simulink model "encoder"  (R2024b)
settings: Solver=FixedStepAuto  StartTime=0.0  StopTime=50  FixedStep=0.1  RelTol=1e-3  EnableMultiTasking=on
libraries: stm32f4xxblockslib x4, stm32g4xxblockslib x3, simulink x2
settings Model: STM32="{\"EncoderBlockForG4\":[{\"ID\":\"encoder:1\"},{\"ID\":\"encoder:3\"},{\"ID\":\"encoder:4\"}],\"DigitalPortRead\":[{\"ID\":\"encoder:8\"},{\"ID\":\"encoder:9\"},{\"ID\":\"encoder:25\"},{\"ID\":\"encoder:32\"}]}"  Creator=FREED  LastModifiedBy=FREED
settings OptimizationCC: DefaultParameterBehavior=Inlined  EnhancedBackFolding=on  PassReuseOutputArgsAs=Individual arguments  ZeroExternalMemoryAtStartup=off  ZeroInternalMemoryAtStartup=off  MaxStackSize=512  OptimizeBlockOrder=speed  DifferentSizesBufferReuse=on  OptimizationCustomize=off  EfficientTunableParamExpr=on
settings DebuggingCC: ParameterTunabilityLossMsg=error
settings HardwareCC: ProdBitPerPointer=32  ProdBitPerSizeT=32  ProdBitPerPtrDiffT=32  ProdLargestAtomicInteger=Long  ProdLargestAtomicFloat=Double  ProdWordSize=32  ProdLongLongMode=on  ProdHWDeviceType=ARM Compatible->ARM Cortex-M
settings SFSimCC: MATLABDynamicMemAlloc=off
settings RTWCC: Description=Embedded Coder  SystemTargetFile=ert.tlc  HardwareBoard=STM32G4xx Based  TemplateMakefile=ert_default_tmf  Toolchain=GNU Tools for ARM Embedded Processors
settings CodeAppCC: ForceParamTrailComments=on  IgnoreCustomStorageClasses=off  OperatorAnnotations=on  SimulinkDataObjDesc=on  SFDataObjDesc=on  InsertBlockDesc=on
settings ERTTargetCC: TargetLangStandard=C99 (ISO)  CodeReplacementLibrary=ARM Cortex-M  ExtModeTransport=3  ExtModeStaticAlloc=on  ExtModeStaticAllocSize=2048  ExtModeMexFile=ext_xcp  ExtModeIntrfLevel=Level2 - Open

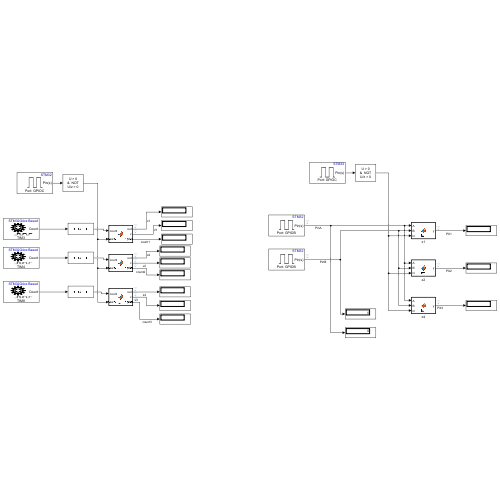
[thumbnail: Simulink's stored preview of the top-level diagram]
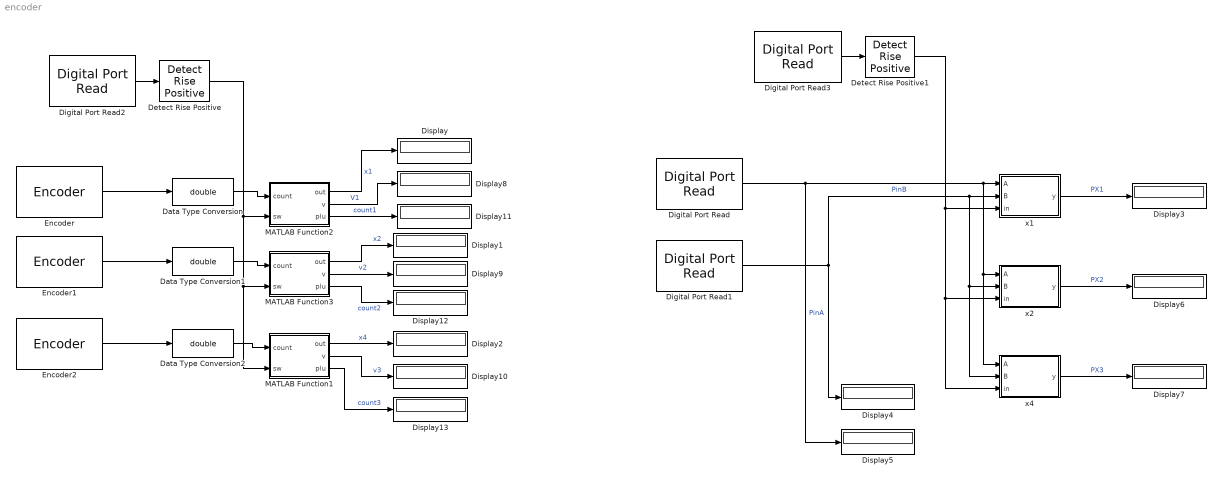
== system encoder ==
  Data Type Conversion : DataTypeConversion  OutDataTypeStr=double  SaturateOnIntegerOverflow=off  RndMeth=Floor
  Data Type Conversion1 : DataTypeConversion  OutDataTypeStr=double  SaturateOnIntegerOverflow=off  RndMeth=Floor
  Data Type Conversion2 : DataTypeConversion  OutDataTypeStr=double  SaturateOnIntegerOverflow=off  RndMeth=Floor
  Detect Rise Positive : simulink/Logic and Bit Operations/Detect Rise Positive  vinit=0  OutDataTypeStr=boolean
  Detect Rise Positive1 : simulink/Logic and Bit Operations/Detect Rise Positive  vinit=0  OutDataTypeStr=boolean
  Digital Port Read : stm32f4xxblockslib/Digital Port Read  PortName=GPIOB  PinNumber=[4]  ReadOperation=on  IOAsArray=on  SampleTime=-1  EnableSimPort=off  hoistedMaskSrc=ECSoC/ECSimCodegen/Digital Port Read
      settings: LibrarySourceBlock=stm32g4xxblockslib/Digital Port Read
  Digital Port Read1 : stm32f4xxblockslib/Digital Port Read  PortName=GPIOB  PinNumber=[5]  ReadOperation=on  IOAsArray=on  SampleTime=-1  EnableSimPort=off  hoistedMaskSrc=ECSoC/ECSimCodegen/Digital Port Read
      settings: LibrarySourceBlock=stm32g4xxblockslib/Digital Port Read
  Digital Port Read2 : stm32f4xxblockslib/Digital Port Read  PortName=GPIOC  PinNumber=[13]  ReadOperation=on  IOAsArray=on  SampleTime=-1  EnableSimPort=off  hoistedMaskSrc=ECSoC/ECSimCodegen/Digital Port Read
      settings: LibrarySourceBlock=stm32g4xxblockslib/Digital Port Read
  Digital Port Read3 : stm32f4xxblockslib/Digital Port Read  PortName=GPIOC  PinNumber=[13]  ReadOperation=on  IOAsArray=on  SampleTime=-1  EnableSimPort=off  hoistedMaskSrc=ECSoC/ECSimCodegen/Digital Port Read
      settings: LibrarySourceBlock=stm32g4xxblockslib/Digital Port Read
  Display{,1..13} (14 alike) : Display
  Encoder : stm32g4xxblockslib/Encoder  TimerModule=TIM3  EnableResetInput=off  OutputCountAfterFirstIndex=off  OutputValidIndex=off  OutputDirection=off  OutputStatus=off  SampleTime=-1
  Encoder1 : stm32g4xxblockslib/Encoder  TimerModule=TIM4  EnableResetInput=off  OutputCountAfterFirstIndex=off  OutputValidIndex=off  OutputDirection=off  OutputStatus=off  SampleTime=-1
  Encoder2 : stm32g4xxblockslib/Encoder  TimerModule=TIM8  EnableResetInput=off  OutputCountAfterFirstIndex=off  OutputValidIndex=off  OutputDirection=off  OutputStatus=off  SampleTime=-1
  MATLAB Function1 : MATLAB Function  TreatAsAtomicUnit=on
  MATLAB Function2 : MATLAB Function  TreatAsAtomicUnit=on
  MATLAB Function3 : MATLAB Function  TreatAsAtomicUnit=on
  x1 : MATLAB Function  TreatAsAtomicUnit=on
  x2 : MATLAB Function  TreatAsAtomicUnit=on
  x4 : MATLAB Function  TreatAsAtomicUnit=on
  wires:
  Digital Port Read1/1 -> Display4/1, x4/2(B), x2/2(B), x1/2(B)  "PinB"
  x1/1(y) -> Display3/1  "PX1"
  Digital Port Read/1 -> Display5/1, x4/1(A), x2/1(A), x1/1(A)  "PinA"
  MATLAB Function2/1(out) -> Display/1  "x1"
  Encoder/1 -> Data Type Conversion/1
  Data Type Conversion/1 -> MATLAB Function2/1(count)
  MATLAB Function1/1(out) -> Display2/1  "x4"
  MATLAB Function3/1(out) -> Display1/1  "x2"
  Data Type Conversion1/1 -> MATLAB Function3/1(count)
  Data Type Conversion2/1 -> MATLAB Function1/1(count)
  Encoder2/1 -> Data Type Conversion2/1
  Encoder1/1 -> Data Type Conversion1/1
  Digital Port Read2/1 -> Detect Rise Positive/1
  Detect Rise Positive/1 -> MATLAB Function1/2(sw), MATLAB Function3/2(sw), MATLAB Function2/2(sw)
  x2/1(y) -> Display6/1  "PX2"
  x4/1(y) -> Display7/1  "PX3"
  Digital Port Read3/1 -> Detect Rise Positive1/1
  Detect Rise Positive1/1 -> x1/3(in), x4/3(in), x2/3(in)
  MATLAB Function2/2(v) -> Display8/1  "V1"
  MATLAB Function3/2(v) -> Display9/1  "v2"
  MATLAB Function1/2(v) -> Display10/1  "v3"
  MATLAB Function2/3(plu) -> Display11/1  "count1"
  MATLAB Function3/3(plu) -> Display12/1  "count2"
  MATLAB Function1/3(plu) -> Display13/1  "count3"

== matlab function encoder/x1 ==
  data: A input; y output; B input; in input
function y = fcn(A,B,in)
persistent c
persistent stageA
if isempty(c)
   c = 0;
   stageA=1;
end
if in == 1 
   c = 0;
end
if A==0 && stageA==1
    stageA=0;
    if B==1
        c=c+1;
    else
        c=c-1;
    end
else
    if A==1
        stageA=1;
    end
end
y = c;

== matlab function encoder/MATLAB Function2 ==
  data: count input; out output; sw input; v output; plu output double
function [out,v,plu] = MATLAB_Function2(count,sw)
persistent pulse
persistent lastpulse
persistent lastrad;
if isempty(pulse)
   pulse= 0;
   lastrad =0;
   lastpulse=0;
   
end
if sw ==1
    pulse=0;
end
    if count>lastpulse
        if (count-lastpulse)>100
            pulse=pulse-(65520-count);
        else
            pulse=pulse+(count-lastpulse);
        end
    else 
       if count<lastpulse
        if (lastpulse-count)>100
            pulse=pulse+(count);
        else
           pulse=pulse-(lastpulse-count);
       end
        end
    end
plu = pulse;
out = pulse*((2*pi)/24);
v= (pulse*((2*pi)/24)-lastrad)/0.1;
lastpulse=count;
lastrad=pulse*((2*pi)/24);

== matlab function encoder/MATLAB Function3 ==
  data: count input; out output; sw input; v output; plu output double
function [out,v,plu] = MATLAB_Function3(count,sw)
persistent pulse
persistent lastpulse
persistent lastrad;
if isempty(pulse)
   pulse= 0;
   lastrad =0;
   lastpulse=0;
   
end
if sw ==1
    pulse=0;
end
    if count>lastpulse
        if (count-lastpulse)>100
            pulse=pulse-(65520-count);
        else
            pulse=pulse+(count-lastpulse);
        end
    else 
       if count<lastpulse
        if (lastpulse-count)>100
            pulse=pulse+(count);
        else
           pulse=pulse-(lastpulse-count);
       end
        end
    end
plu = pulse;
out = pulse*((2*pi)/48);
v= (pulse*((2*pi)/48)-lastrad)/0.1;
lastpulse=count;
lastrad=pulse*((2*pi)/48);

== matlab function encoder/MATLAB Function1 ==
  data: count input; out output; sw input; v output; plu output double
function [out,v,plu] = MATLAB_Function1(count,sw)
persistent pulse
persistent lastpulse
persistent lastrad;
if isempty(pulse)
   pulse= 0;
   lastrad =0;
   lastpulse=0;
   
end
if sw ==1
    pulse=0;
end
    if count>lastpulse
        if (count-lastpulse)>100
            pulse=pulse-(65520-count);
        else
            pulse=pulse+(count-lastpulse);
        end
    else 
       if count<lastpulse
        if (lastpulse-count)>100
            pulse=pulse+(count);
        else
           pulse=pulse-(lastpulse-count);
       end
        end
    end
plu = pulse;
out = pulse*((2*pi)/96);
v= (pulse*((2*pi)/96)-lastrad)/0.1;
lastpulse=count;
lastrad=pulse*((2*pi)/96);

== matlab function encoder/x2 ==
  data: A input; y output; B input; in input
function y = fcn(A,B,in)
persistent c
persistent stageA
if isempty(c)
   c = 0;
   stageA=1;
end
if in == 1 
   c = 0;
end
if A==0 && stageA==1
    stageA=0;
    if B==1
        c=c+1;
    else
        c=c-1;
    end
else
    if A==1 && stageA ==0 
        stageA=1;
        if B==0
            c=c+1;
        else
            c=c-1;
        end
    end
end
y = c;

== matlab function encoder/x4 ==
  data: A input; y output; B input; in input
function y = fcn(A,B,in)
persistent c
persistent stageA
persistent stageB
if isempty(c)
   c = 0;
   stageA=1;
   stageB=1;
end
if in==1
    c=0;
end
if A==0 && stageA==1
    stageA=0;
    if B==1
        c=c+1;
    else
        c=c-1;
    end
else
    if A==1 && stageA==0
        stageA=1;
        if B==0
            c=c+1;
        else
            c=c-1;
        end
    end
end

if B==0 && stageB==1
    stageB=0;
    if A==0
        c=c+1;
    else
        c=c-1;
    end
else
    if B==1 && stageB==0
        stageB=1;
        if A==1
            c=c+1;
        else
            c=c-1;
        end
    end
end


y = c;
